simulink model "speed_torque_theta_v1_2"  (R2021a)
settings: Solver=VariableStepAuto  StartTime=0.0  StopTime=10.0  RelTol=1e-3
libraries: eeTransforms x2
settings Model: Creator=danesh  LastModifiedBy=danesh

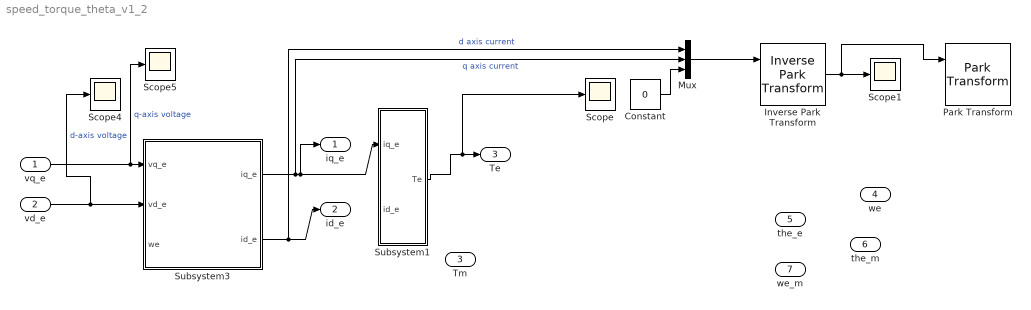
== system speed_torque_theta_v1_2 ==
  vq_e : Inport
  vd_e : Inport  Port=2
  Tm : Inport  Port=3
  Constant : Constant  Value=0
  Inverse Park Transform : eeTransforms/Inverse Park Transform  AxisAlignment=Q-axis  PowerInvariant=off
  Mux : Mux  Inputs=3
  Park Transform : eeTransforms/Park Transform  AxisAlignment=Q-axis  PowerInvariant=off
  Scope{,1,4..5} (4 alike) : Scope
  Subsystem1 : Subsystem
  Subsystem3 : Subsystem
  iq_e : Outport  VectorParamsAs1DForOutWhenUnconnected=off
  id_e : Outport  Port=2  VectorParamsAs1DForOutWhenUnconnected=off
  Te : Outport  Port=3  VectorParamsAs1DForOutWhenUnconnected=off
  we : Outport  Port=4  VectorParamsAs1DForOutWhenUnconnected=off
  the_e : Outport  Port=5  VectorParamsAs1DForOutWhenUnconnected=off
  the_m : Outport  Port=6  VectorParamsAs1DForOutWhenUnconnected=off
  we_m : Outport  Port=7  VectorParamsAs1DForOutWhenUnconnected=off
  wires:
  Subsystem1/1(Te) -> Scope/1, Te/1
  Mux/1 -> Inverse Park Transform/1
  Subsystem3/2(id_e) -> Mux/1, id_e/1  "d axis current"
  Inverse Park Transform/1 -> Park Transform/1, Scope1/1
  vq_e/1 -> Scope5/1, Subsystem3/1(vq_e)  "q-axis voltage"
  Constant/1 -> Mux/3
  Subsystem3/1(iq_e) -> Mux/2, Subsystem1/1(iq_e), iq_e/1  "q axis current"
  vd_e/1 -> Scope4/1, Subsystem3/2(vd_e)  "d-axis voltage"

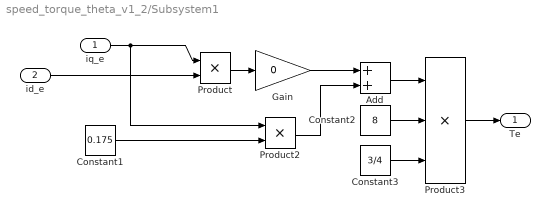
== system speed_torque_theta_v1_2/Subsystem1 ==
  iq_e : Inport
  id_e : Inport  Port=2
  Add : Sum
  Constant1 : Constant  Value=0.175
  Constant2 : Constant  Value=8
  Constant3 : Constant  Value=3/4
  Gain : Gain  Gain=0
  Product : Product  RndMeth=Zero
  Product2 : Product  RndMeth=Zero
  Product3 : Product  Inputs=3  RndMeth=Zero
  Te : Outport  VectorParamsAs1DForOutWhenUnconnected=off
  wires:
  iq_e/1 -> Product/1, Product2/1
  id_e/1 -> Product/2
  Product/1 -> Gain/1
  Constant1/1 -> Product2/2
  Gain/1 -> Add/1
  Product2/1 -> Add/2
  Add/1 -> Product3/1
  Constant2/1 -> Product3/2
  Constant3/1 -> Product3/3
  Product3/1 -> Te/1

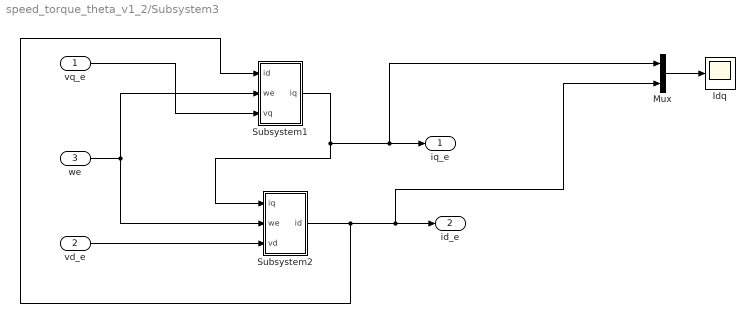
== system speed_torque_theta_v1_2/Subsystem3 ==
  vq_e : Inport
  vd_e : Inport  Port=2
  we : Inport  Port=3
  Idq : Scope
  Mux : Mux  Inputs=2
  Subsystem1 : Subsystem
  Subsystem2 : Subsystem
  iq_e : Outport  VectorParamsAs1DForOutWhenUnconnected=off
  id_e : Outport  Port=2  VectorParamsAs1DForOutWhenUnconnected=off
  wires:
  vq_e/1 -> Subsystem1/3(vq)
  vd_e/1 -> Subsystem2/3(vd)
  we/1 -> Subsystem1/2(we), Subsystem2/2(we)
  Subsystem1/1(iq) -> Subsystem2/1(iq), Mux/1, iq_e/1
  Subsystem2/1(id) -> Subsystem1/1(id), Mux/2, id_e/1
  Mux/1 -> Idq/1

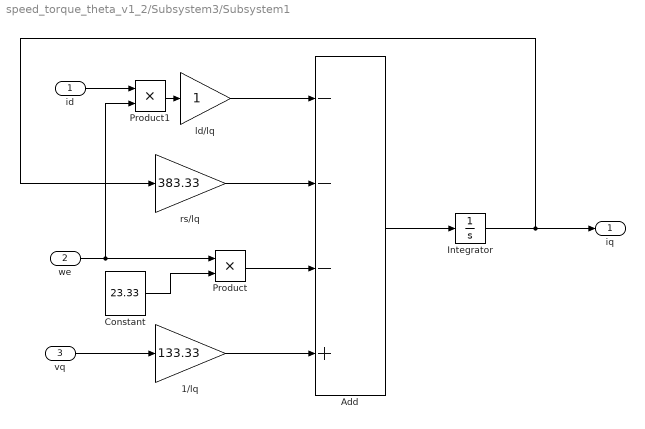
== system speed_torque_theta_v1_2/Subsystem3/Subsystem1 ==
  id : Inport
  we : Inport  Port=2
  vq : Inport  Port=3
  "1/lq " : Gain  Gain=133.33
  Add : Sum  Inputs=---+
  Constant : Constant  Value=23.33
  Integrator : Integrator
  Product : Product  RndMeth=Zero
  Product1 : Product  RndMeth=Zero
  "ld/lq " : Gain
  rs/lq : Gain  Gain=383.33
  iq : Outport  VectorParamsAs1DForOutWhenUnconnected=off
  wires:
  vq/1 -> "1/lq "/1
  "ld/lq "/1 -> Add/1
  rs/lq/1 -> Add/2
  "1/lq "/1 -> Add/4
  Add/1 -> Integrator/1
  Integrator/1 -> rs/lq/1, iq/1
  Product/1 -> Add/3
  we/1 -> Product/1, Product1/2
  Constant/1 -> Product/2
  Product1/1 -> "ld/lq "/1
  id/1 -> Product1/1

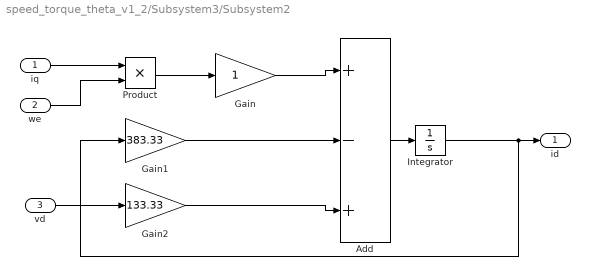
== system speed_torque_theta_v1_2/Subsystem3/Subsystem2 ==
  iq : Inport
  we : Inport  Port=2
  vd : Inport  Port=3
  Add : Sum  Inputs=+-+
  Gain : Gain
  Gain1 : Gain  Gain=383.33
  Gain2 : Gain  Gain=133.33
  Integrator : Integrator
  Product : Product  RndMeth=Zero
  id : Outport  VectorParamsAs1DForOutWhenUnconnected=off
  wires:
  iq/1 -> Product/1
  we/1 -> Product/2
  Product/1 -> Gain/1
  Gain/1 -> Add/1
  Add/1 -> Integrator/1
  Gain1/1 -> Add/2
  vd/1 -> Gain2/1
  Gain2/1 -> Add/3
  Integrator/1 -> Gain1/1, id/1
